simulink subsystem "LQRmotor"  (R2024a)
settings: Solver=VariableStepAuto  StartTime=0.0  StopTime=10.0  RelTol=1e-3
undefined symbols (not defined in the file or in its folder): K_aug_lqr
settings Model: Creator=Peter  LastModifiedBy=Peter

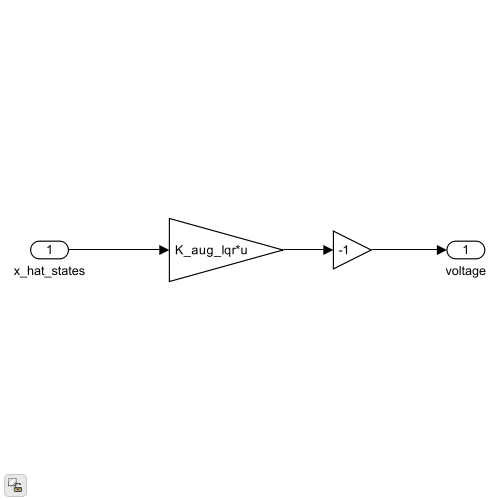
[thumbnail: Simulink's stored preview of the top-level diagram]
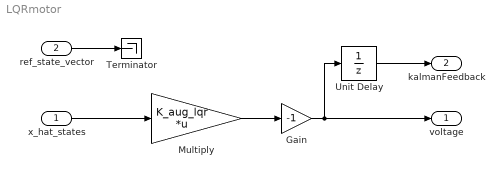
== system LQRmotor ==
  x_hat_states : Inport
  ref_state_vector : Inport  Port=2
  Gain : Gain  Gain=-1
  Multiply : Gain  Gain=K_aug_lqr  Multiplication=Matrix(K*u)
  Terminator : Terminator
  Unit Delay : UnitDelay  SampleTime=-1  HasFrameUpgradeWarning=on
  voltage : Outport
  kalmanFeedback : Outport  Port=2  OutDataTypeStr=single
  wires:
  Gain/1 -> voltage/1, Unit Delay/1
  x_hat_states/1 -> Multiply/1
  Multiply/1 -> Gain/1
  Unit Delay/1 -> kalmanFeedback/1
  ref_state_vector/1 -> Terminator/1
